simulink model "IIR_Filter_Design"  (R2023a)
settings: Solver=FixedStepDiscrete  StartTime=0.0  StopTime=Inf  RelTol=1e-3  EnableMultiTasking=on
undefined symbols (not defined in the file): fdesignblkfcn, gcbh
libraries: dspsrcs4 x2, dsparch4 x1, dspfdesign x1
settings Model: ModifiedByFormat=The MathWorks Inc.  Creator=The MathWorks, Inc.  LastModifiedBy=The MathWorks Inc.
settings SolverCC: AlgebraicLoopSolver=TrustRegion
settings DataIOCC: LimitDataPoints=on  SaveFormat=Array  SaveOutput=off  SignalLogging=off  DSMLogging=off  SaveTime=off  ReturnWorkspaceOutputs=off
settings OptimizationCC: DefaultParameterBehavior=Inlined  EnhancedBackFolding=on  PassReuseOutputArgsAs=Individual arguments  ZeroExternalMemoryAtStartup=off  ZeroInternalMemoryAtStartup=off  OptimizeBlockOrder=speed  DifferentSizesBufferReuse=on  OptimizationCustomize=off  EfficientTunableParamExpr=on
settings DebuggingCC: SolverPrmCheckMsg=warning  ParameterTunabilityLossMsg=error  UnconnectedInputMsg=warning  UnconnectedOutputMsg=warning  UnconnectedLineMsg=warning  AllowSymbolicDim=off  SFUnexpectedBacktrackingDiag=warning  SFNoUnconditionalDefaultTransitionDiag=warning  SFExecutionAtInitializationDiag=none  ArithmeticOperatorsInVariantConditions=warning
settings HardwareCC: ProdBitPerPointer=32  ProdBitPerSizeT=32  ProdBitPerPtrDiffT=32  ProdLargestAtomicFloat=None  ProdIntDivRoundTo=Undefined  ProdEndianess=Unspecified  ProdWordSize=32  ProdHWDeviceType=32-bit Generic
settings ModelReferenceCC: EnableRefExpFcnMdlSchedulingChecks=on  PropagateSignalLabelsOutOfModel=off
settings SFSimCC: SimUseLocalCustomCode=off  MATLABDynamicMemAlloc=off  CustomCodeUndefinedFunction=UseInterfaceOnly
settings RTWCC: Description=Embedded Coder  SystemTargetFile=ert.tlc  GenCodeOnly=on  TemplateMakefile=ert_default_tmf  RTWUseLocalCustomCode=off  DLArmComputeVersion=19.05
settings CodeAppCC: ForceParamTrailComments=on  IgnoreCustomStorageClasses=off  OperatorAnnotations=on  SimulinkDataObjDesc=on  SFDataObjDesc=on  InsertBlockDesc=on
settings ERTTargetCC: GenerateSampleERTMain=on  InlinedParameterPlacement=NonHierarchical  ERTCustomFileTemplate=example_file_process.tlc
settings ConfigComp: CovMetricSettings=dw  CovSaveCumulativeToWorkspaceVar=on  CovSaveSingleToWorkspaceVar=on  CovExternalEMLEnable=off  CovSFcnEnable=off

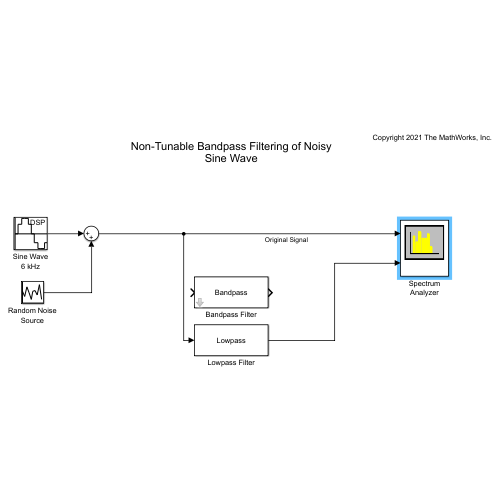
[thumbnail: Simulink's stored preview of the top-level diagram]
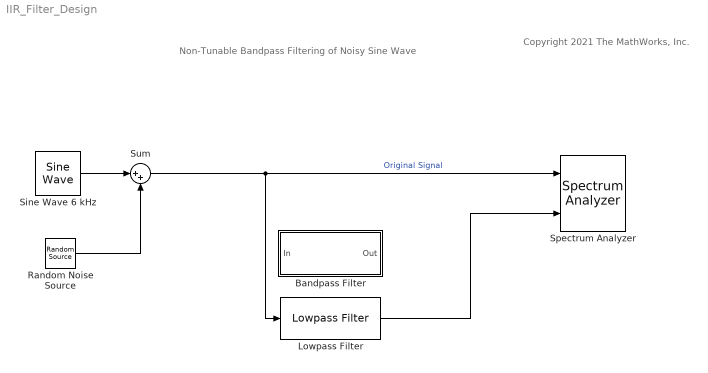
== system IIR_Filter_Design ==
  note: Non-Tunable Bandpass Filtering of Noisy Sine Wave
  note: Copyright 2021 The MathWorks, Inc.
  Bandpass Filter : Subsystem  DialogController=fdesignblkfcn  InitFcn=fdesignblkfcn(gcbh, {'InitFcn'});  mask(Bandpass Filter){}
      mask help: Design a bandpass filter
      settings: CopyFcn=fdesignblkfcn(gcbh, {'CopyFcn'});
      mask Help: helpview(mapfilelocation('dsp'), 'dspbandpassfilter');
      mask Display: disp('Bandpass');
  Lowpass Filter : dspfdesign/Lowpass Filter  FilterType=IIR  DesignForMinimumOrder=on  FilterOrder=50  PassbandFrequency=6000  StopbandFrequency=6500  PassbandRipple=0.1  StopbandAttenuation=80  SampleRateMode=Specify on dialog  SampleRate=44100  SimulateUsing=Interpreted execution  roundingMode=Floor  coeffsDataTypeStr=fixdt(1,16)
  Random Noise Source : dspsrcs4/Random Source  SrcType=Gaussian  NormMethod=Ziggurat  CltLength=12  MinVal=0  MaxVal=1  MeanVal=0  VarVal=1e-5  RepMode=Specify seed  rawSeed=3  IsInherit=off  SampMode=Discrete  SampTime=1/44100  SampFrame=1024  DataType=Double  OutComplex=Real  OutputFrames=off
  Sine Wave 6 kHz : dspsrcs4/Sine Wave  Amplitude=1  Frequency=6000  Phase=0  SampleMode=Discrete  OutComplex=Real  CompMethod=Trigonometric fcn  TableSize=Speed  SampleTime=1/44100  SamplesPerFrame=1024  ResetState=Restart at time zero  OutputFrames=off  dataType=double  wordLen=16  udDataType=sfix(16)  fracBitsMode=Best precision  numFracBits=15  OutDataTypeStr=double  LastOutDataTypeStr=double
  Spectrum Analyzer : SpectrumAnalyzer  NumInputPorts=2  WindowPosition=[170.000000,83.000000,1191.000000,661.000000,]  ScopeFrameLocation=window  Method=Welch  SampleRate=44100  PlotAsTwoSidedSpectrum=off  AxesScaling=Manual  Span=44100  StartFrequency=-22050  StopFrequency=22050  FrequencyResolutionMethod=Window length  AveragingMethod=Exponential  Title=Power spectrum of original v/s filtered signal  YLimits=[-129.19542001644344964,43.218788306243240527]  ShowLegend=on  ChannelNames="[\"Original Signal\",\"Filtered Signal\"]"  DefaultConfigurationName=spbscopes.SpectrumAnalyzerBlockCfg  IsFrequencyInputMode=0  FrequencyVectorPort=0  FrequencyVectorFromPort=0  FrequencyInputRBWPort=0  FrequencyInputRBWFromPort=0
      settings: OpenAtSimulationStart=off
  Sum : Sum  Inputs=|++
  wires:
  Sum/1 -> Lowpass Filter/1, Spectrum Analyzer/1  "Original Signal"
  Sine Wave 6 kHz/1 -> Sum/1
  Random Noise Source/1 -> Sum/2
  Lowpass Filter/1 -> Spectrum Analyzer/2

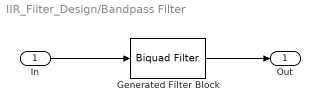
== system IIR_Filter_Design/Bandpass Filter ==
  In : Inport
  Generated Filter Block : dsparch4/Biquad Filter  Tag=BlockMethodSubSystem  FilterSource=Dialog parameters  CoeffSource=Specify via dialog  FilterObject=BQF  IIRFiltStruct=Direct form II  BiQuadCoeffs=[0.125869297016915377 0 -0.125869297016915377 1 -1.34390546472826866 0.915040749018974031;0.0656121180375594387 0 -0.0656121180375594387 1 -1.16122268541534979 0.905887423904348066;0.0849285957057947793 0 -0.0849285957057947793 1 -1.27123473799067255 0.870050693199404312;0.0185985573206114384 0 -0.0185985573206114384 1 -1.18347367375318724 0.863601262984001083;0.159605087222613434 0 -0.159605087222613434 1 -1.41043725076161142 0.981451841259691315;0.0600295830172420594 0 -0.0600295830172420594 1 -1.18035427365937795 0.978832212264976409;0.131232435799951502 0 -0.131232435799951502 1 -1.30744608465992096 0.889179780611041748;0.0897246573019897797 0 -0.0897246573019897797 1 -1.16761887258936792 0.880233509308278705;0.0757281400770920404 0 -0.0757281400770920404 1 -1.2371804000830291 0.85884235496636685;0.0366761055638505154 0 -0.0366761055638505154 1 -1.20726901956567767 0.856499733572212874;0.145182340958319667 0 -0.145182340958319667 1 -1.37880997391524152 0.94628865549389285;0.700444398540468249 0 -0.700444398540468249 1 -1.1653322667715198 0.939384311325326515]  ScaleValues=[0.0604683256900894403;1;1;1;1;1;1;1;1;1;1;1;1]  IC=0  ICnum=0  ICden=0  a0Flag=Warning  optimizeScaleValues=off  ScaleValueMode=Specify via input port (g)  InputProcessing=Columns as channels (frame based)  roundingMode=Floor  overflowMode=off  scaleValueFracLength=14  denProdOutputFracLength=30  denAccumFracLength=30  secondMemoryFracLength=15
  Out : Outport  VectorParamsAs1DForOutWhenUnconnected=off
  wires:
  In/1 -> Generated Filter Block/1
  Generated Filter Block/1 -> Out/1
